simulink model "LabosimuladoPID"  (R2025b)
settings: Solver=VariableStepAuto  StartTime=0.0  StopTime=60  RelTol=1e-3
values from neighbouring files (symbols this model uses):
  ss4 = ss(tf1)    [pruebassytflabo2parte3.m]
  X0 = [0 0 0 0]    [PIDworkspace.mat]    (also in pruebassytflabo2parte3.m = [0;0;0;0])
undefined symbols (not defined in the file or in its folder): ss1
settings Model: Creator=Froilán Pardo  LastModifiedBy=Froilán Pardo

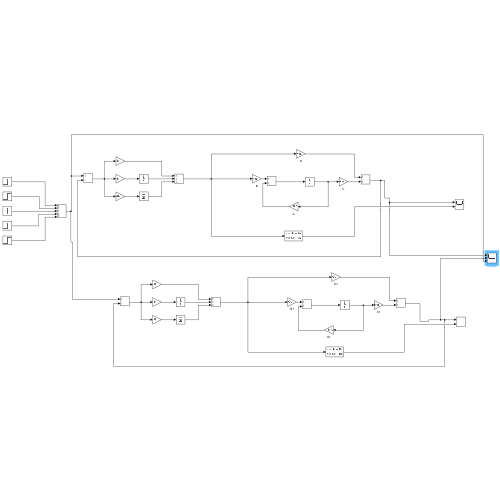
[thumbnail: Simulink's stored preview of the top-level diagram]
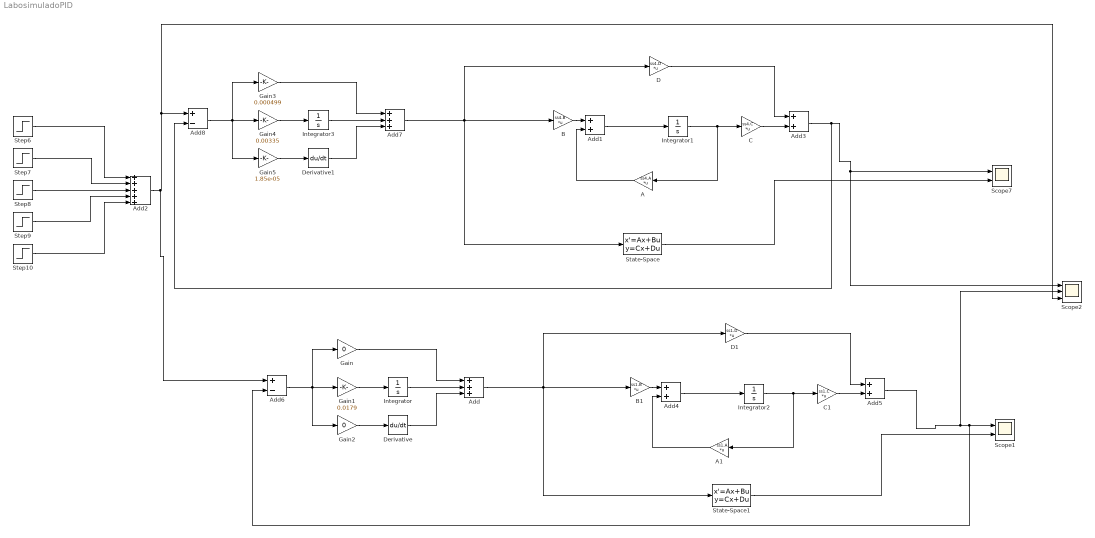
== system LabosimuladoPID ==
  A : Gain  Gain=ss4.A  Multiplication=Matrix(K*u)
  A1 : Gain  Gain=ss1.A  Multiplication=Matrix(K*u)
  Add : Sum  Inputs=+++
  Add{1,3..5} (4 alike) : Sum
  Add2 : Sum  Inputs=+++++
  Add6 : Sum  Inputs=+-
  Add7 : Sum  Inputs=+++
  Add8 : Sum  Inputs=+-
  B : Gain  Gain=ss4.B  Multiplication=Matrix(K*u)
  B1 : Gain  Gain=ss1.B  Multiplication=Matrix(K*u)
  C : Gain  Gain=ss4.C  Multiplication=Matrix(K*u)
  C1 : Gain  Gain=ss1.C  Multiplication=Matrix(K*u)
  D : Gain  Gain=ss4.D  Multiplication=Matrix(K*u)
  D1 : Gain  Gain=ss1.D  Multiplication=Matrix(K*u)
  Derivative : Derivative
  Derivative1 : Derivative
  Gain : Gain  Gain=0
  Gain1 : Gain  Gain=0.0179
  Gain2 : Gain  Gain=0
  Gain3 : Gain  Gain=0.000499
  Gain4 : Gain  Gain=0.00335
  Gain5 : Gain  Gain=1.85e-05
  Integrator : Integrator
  Integrator1 : Integrator  InitialCondition=X0
  Integrator2 : Integrator  InitialCondition=X0
  Integrator3 : Integrator
  Scope1 : Scope  NumInputPorts=2
      settings: ActiveDisplayYMinimum=-0.12512726316876521  ActiveDisplayYMaximum=1.1261453685188871
  Scope2 : Scope  NumInputPorts=3
      settings: ActiveDisplayYMinimum=-0.12588297767957302  ActiveDisplayYMaximum=1.1329467991161575
  Scope7 : Scope  NumInputPorts=2
      settings: ActiveDisplayYMinimum=-0.12588297767957302  ActiveDisplayYMaximum=1.1329467991161575  DataLoggingVariableName=ScopeData7
  State-Space : StateSpace  A=ss4.A  B=ss4.B  C=ss4.C  D=ss4.D  InitialCondition=X0
  State-Space1 : StateSpace  A=ss1.A  B=ss1.B  C=ss1.C  D=ss1.D  InitialCondition=X0
  Step10 : Step  Time=48  After=0.2  SampleTime=0
  Step6 : Step  Time=0  After=0.2  SampleTime=0
  Step7 : Step  Time=12  After=0.2  SampleTime=0
  Step8 : Step  Time=24  After=0.2  SampleTime=0
  Step9 : Step  Time=36  After=0.2  SampleTime=0
  wires:
  Step6/1 -> Add2/1
  Step9/1 -> Add2/4
  Step7/1 -> Add2/2
  Step10/1 -> Add2/5
  Step8/1 -> Add2/3
  Integrator1/1 -> C/1, A/1
  B/1 -> Add1/1
  D/1 -> Add3/1
  C/1 -> Add3/2
  State-Space/1 -> Scope7/2
  A/1 -> Add1/2
  Add1/1 -> Integrator1/1
  C1/1 -> Add5/2
  B1/1 -> Add4/1
  Add4/1 -> Integrator2/1
  Integrator2/1 -> C1/1, A1/1
  D1/1 -> Add5/1
  Add5/1 -> Scope2/2, Add6/2, Scope1/1
  State-Space1/1 -> Scope1/2
  A1/1 -> Add4/2
  Add/1 -> State-Space1/1, B1/1, D1/1
  Derivative/1 -> Add/3
  Gain2/1 -> Derivative/1
  Integrator/1 -> Add/2
  Gain1/1 -> Integrator/1
  Gain/1 -> Add/1
  Add6/1 -> Gain/1, Gain1/1, Gain2/1
  Add8/1 -> Gain3/1, Gain4/1, Gain5/1
  Gain3/1 -> Add7/1
  Add3/1 -> Add8/2, Scope2/1, Scope7/1
  Gain4/1 -> Integrator3/1
  Derivative1/1 -> Add7/3
  Integrator3/1 -> Add7/2
  Add7/1 -> State-Space/1, D/1, B/1
  Gain5/1 -> Derivative1/1
  Add2/1 -> Add6/1, Add8/1, Scope2/3
